simulink model "slturtlesim_control"  (R2021b)
settings: Solver=FixedStepAuto  StartTime=0.0  StopTime=Inf  RelTol=1e-3
undefined symbols (not defined in the file): angular, Call, Function, linear, theta, x, y
libraries: ros2lib x4, simulink x1, mobileRoboticsLib x1
settings Model: Creator=beave  LastModifiedBy=beave
settings OptimizationCC: EnhancedBackFolding=on  PassReuseOutputArgsAs=Individual arguments  ZeroExternalMemoryAtStartup=off  ZeroInternalMemoryAtStartup=off  MaxStackSize=64  OptimizeBlockOrder=speed  DifferentSizesBufferReuse=on  OptimizationCustomize=off  EfficientTunableParamExpr=on
settings DebuggingCC: ParameterTunabilityLossMsg=error
settings SFSimCC: MATLABDynamicMemAlloc=off
settings RTWCC: Description=Embedded Coder  SystemTargetFile=ert.tlc  HardwareBoard=Robot Operating System 2 (ROS 2)  TemplateMakefile=ert_default_tmf  Toolchain=Colcon Tools  TargetLang=C++
settings CodeAppCC: ForceParamTrailComments=on  IgnoreCustomStorageClasses=off  OperatorAnnotations=on  SimulinkDataObjDesc=on  SFDataObjDesc=on  InsertBlockDesc=on
settings ERTTargetCC: CodeInterfacePackaging=C++ class  SupportContinuousTime=on  RootIOFormat=Structure reference

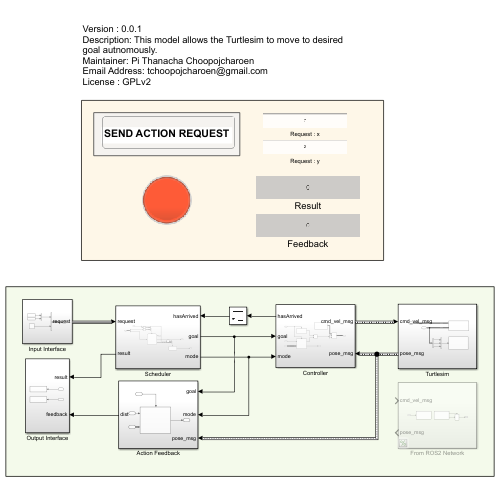
[thumbnail: Simulink's stored preview of the top-level diagram]
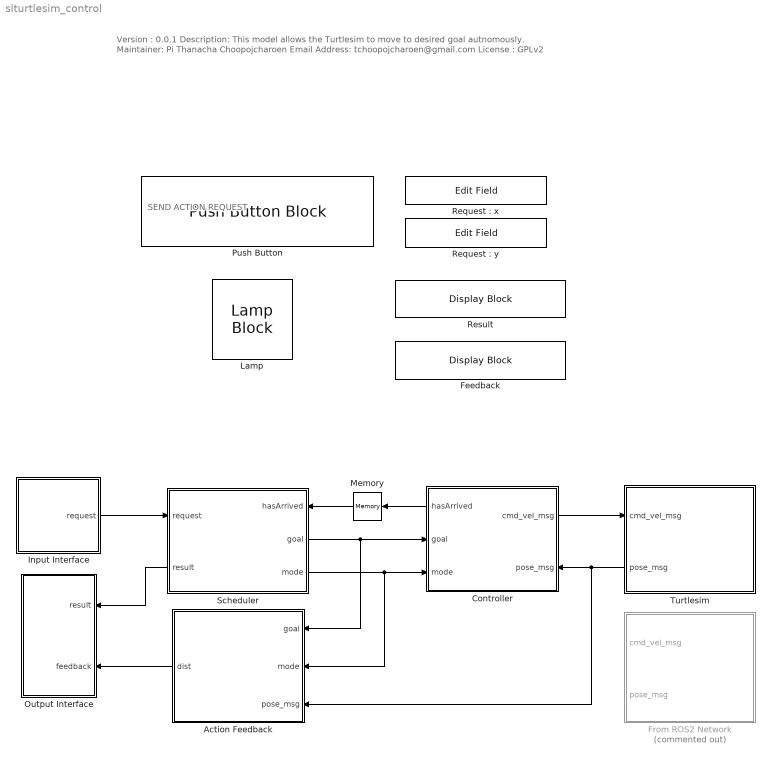
== system slturtlesim_control ==
  note: Version : 0.0.1
      | Description: This model allows the Turtlesim to move to desired goal autnomously.
      | Maintainer: Pi Thanacha Choopojcharoen
      | Email Address: tchoopojcharoen@gmail.com
      | License : GPLv2
  note: SEND ACTION REQUEST
  Action Feedback : Subsystem
      settings: PortSchema="{\"entries\":[{\"content\":{\"sides\":[{\"content\":{\"connectorIds\":[\"Out1\"]},\"type\":\"ConnectorPlacement.EquallySpacedRectSide\",\"uuid\":\"16802256-551c-4223-bfc5-a76a4b41f33f\"},{\"content\":{\"connectorIds\":[\"In1\",\"In2\",\"In3\"],\"side\":\"RIGHT\"},\"type\":\"ConnectorPlacement.EquallySpacedRectSide\",\"uuid\":\"5606428e-27b0-4fd9-928f-2a9a8baead9b\"},{\"content\":{\"connectorIds\":[],\"side\":\"TOP\"},\"type\":\"ConnectorPlacement.EquallySpacedRectSide\",\"uuid\":\"29cf616f-a397-4c6b-9e61-c1bdda273a98\"}]},\"type\":\"ConnectorPlacement.EquallySpacedConnector\",\"uuid\":\"ad2a9b87-c534-416c-adde-7d63bbec43f7\"}],\"packageUris\":[\"http://schema.mathworks.com/mf0/Connector/R2020b\"],\"version\":\"1.0\"}"
  Controller : Subsystem
      settings: PortSchema="{\"entries\":[{\"content\":{\"sides\":[{\"content\":{\"connectorIds\":[\"Out2\",\"In1\",\"In2\"]},\"type\":\"ConnectorPlacement.EquallySpacedRectSide\",\"uuid\":\"038c2229-5bef-4150-bdd4-e0d53c992ca9\"},{\"content\":{\"connectorIds\":[\"Out1\",\"In3\"],\"side\":\"RIGHT\"},\"type\":\"ConnectorPlacement.EquallySpacedRectSide\",\"uuid\":\"f3336771-d94a-4ec8-8106-6e13fcccc0ae\"},{\"content\":{\"connectorIds\":[],\"side\":\"TOP\"},\"type\":\"ConnectorPlacement.EquallySpacedRectSide\",\"uuid\":\"c9d4cbcf-6a2f-41c3-9d97-35a13869506d\"},{\"content\":{\"connectorIds\":[],\"side\":\"BOTTOM\"},\"type\":\"ConnectorPlacement.EquallySpacedRectSide\",\"uuid\":\"fffd547c-1bb9-4cdd-bfe2-128d74787c10\"}]},\"type\":\"ConnectorPlacement.EquallySpacedConnector\",\"uuid\":\"42e11a89-ad8d-483b-9082-68cf3f59b49f\"}],\"packageUris\":[\"http://schema.mathworks.com/mf0/Connector/R2020b\"],\"version\":\"1.0\"}"
  Feedback : DisplayBlock  LabelPosition=Hide  Format=short  Transparency=1
  From ROS2 Network : Subsystem  Commented=on
      settings: PortSchema="{\"entries\":[{\"content\":{\"sides\":[{\"content\":{\"connectorIds\":[\"In1\",\"Out1\"]},\"type\":\"ConnectorPlacement.EquallySpacedRectSide\",\"uuid\":\"f269cb0f-6751-420c-b024-d2e3796ade5b\"},{\"content\":{\"connectorIds\":[],\"side\":\"RIGHT\"},\"type\":\"ConnectorPlacement.EquallySpacedRectSide\",\"uuid\":\"2b43efcf-3102-43c3-9588-0e0fabe7b77d\"},{\"content\":{\"connectorIds\":[],\"side\":\"TOP\"},\"type\":\"ConnectorPlacement.EquallySpacedRectSide\",\"uuid\":\"af694c79-adb9-467b-a06b-a7c95e051029\"}]},\"type\":\"ConnectorPlacement.EquallySpacedConnector\",\"uuid\":\"1952be18-0165-4d1b-9c7c-2327e5c332ed\"}],\"packageUris\":[\"http://schema.mathworks.com/mf0/Connector/R2020b\"],\"version\":\"1.0\"}"
  Input Interface : Subsystem
  Lamp : LampBlock  LabelPosition=Hide
  Memory : Memory  InitialCondition=1
  Output Interface : Subsystem
  Push Button : PushButtonBlock  Opacity=0  IconAlignment=Center  IconColor=On  OffValue=0.000000
  "Request : x" : EditField  LabelPosition=Hide  ShowInitialText=on  Alignment=Center
  "Request : y" : EditField  LabelPosition=Hide  ShowInitialText=on  Alignment=Center
  Result : DisplayBlock  LabelPosition=Hide  Format=short  Transparency=1
  Scheduler : Subsystem
      settings: PortSchema="{\"entries\":[{\"content\":{\"sides\":[{\"content\":{\"connectorIds\":[\"In1\",\"Out3\"]},\"type\":\"ConnectorPlacement.EquallySpacedRectSide\",\"uuid\":\"1630b4b1-4c51-4b39-8ddc-aa89298d57f7\"},{\"content\":{\"connectorIds\":[\"In2\",\"Out1\",\"Out2\"],\"side\":\"RIGHT\"},\"type\":\"ConnectorPlacement.EquallySpacedRectSide\",\"uuid\":\"26eab6e1-3412-432a-b46d-5233f76b34aa\"},{\"content\":{\"connectorIds\":[],\"side\":\"TOP\"},\"type\":\"ConnectorPlacement.EquallySpacedRectSide\",\"uuid\":\"460729cf-3c40-4892-baa8-6e87916f7267\"}]},\"type\":\"ConnectorPlacement.EquallySpacedConnector\",\"uuid\":\"4b48c5f2-6058-4723-aff1-2a33b1e01132\"}],\"packageUris\":[\"http://schema.mathworks.com/mf0/Connector/R2020b\"],\"version\":\"1.0\"}"
  Turtlesim : Subsystem
      settings: PortSchema="{\"entries\":[{\"content\":{\"sides\":[{\"content\":{\"connectorIds\":[\"In1\",\"Out1\"]},\"type\":\"ConnectorPlacement.EquallySpacedRectSide\",\"uuid\":\"f269cb0f-6751-420c-b024-d2e3796ade5b\"},{\"content\":{\"connectorIds\":[],\"side\":\"RIGHT\"},\"type\":\"ConnectorPlacement.EquallySpacedRectSide\",\"uuid\":\"2b43efcf-3102-43c3-9588-0e0fabe7b77d\"},{\"content\":{\"connectorIds\":[],\"side\":\"TOP\"},\"type\":\"ConnectorPlacement.EquallySpacedRectSide\",\"uuid\":\"af694c79-adb9-467b-a06b-a7c95e051029\"}]},\"type\":\"ConnectorPlacement.EquallySpacedConnector\",\"uuid\":\"1952be18-0165-4d1b-9c7c-2327e5c332ed\"}],\"packageUris\":[\"http://schema.mathworks.com/mf0/Connector/R2020b\"],\"version\":\"1.0\"}"
  wires:
  Controller/2(hasArrived) -> Memory/1
  Scheduler/1(goal) -> Action Feedback/1(goal), Controller/1(goal)
  Scheduler/2(mode) -> Action Feedback/2(mode), Controller/2(mode)
  Memory/1 -> Scheduler/2(hasArrived)
  Turtlesim/1(pose_msg) -> Action Feedback/3(pose_msg), Controller/3(pose_msg)
  Controller/1(cmd_vel_msg) -> Turtlesim/1(cmd_vel_msg)
  Scheduler/3(result) -> Output Interface/1(result)
  Action Feedback/1(dist) -> Output Interface/2(feedback)
  Input Interface/1(request) -> Scheduler/1(request)

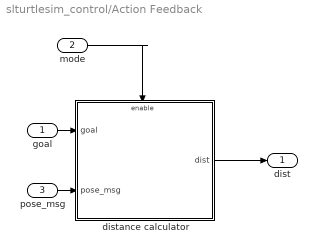
== system slturtlesim_control/Action Feedback ==
  goal : Inport
  mode : Inport  Port=2
  pose_msg : Inport  Port=3
  distance calculator : Subsystem
  dist : Outport
  wires:
  distance calculator/1(dist) -> dist/1
  pose_msg/1 -> distance calculator/2(pose_msg)
  goal/1 -> distance calculator/1(goal)
  mode/1 -> distance calculator/Enable

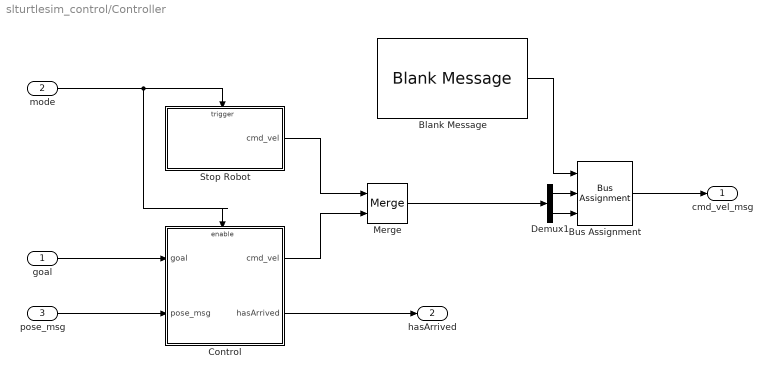
== system slturtlesim_control/Controller ==
  goal : Inport
  mode : Inport  Port=2
  pose_msg : Inport  Port=3
  Blank Message : ros2lib/Blank Message  messageClass=Message  entityType=geometry_msgs/Twist  messageType=geometry_msgs/Twist  SampleTime=inf
      settings: SourceProductBaseCode=RR
  Bus Assignment : BusAssignment  AssignedSignals=linear.x,angular.z
  Control : Subsystem
  Demux1 : Demux  Outputs=2
  Merge : Merge  InitialOutput=[0;0]
  Stop Robot : Subsystem
  cmd_vel_msg : Outport
  hasArrived : Outport  Port=2
  wires:
  pose_msg/1 -> Control/2(pose_msg)
  Control/2(hasArrived) -> hasArrived/1
  goal/1 -> Control/1(goal)
  mode/1 -> Control/Enable, Stop Robot/Trigger
  Control/1(cmd_vel) -> Merge/2
  Stop Robot/1(cmd_vel) -> Merge/1
  Blank Message/1 -> Bus Assignment/1
  Demux1/1 -> Bus Assignment/2
  Demux1/2 -> Bus Assignment/3
  Merge/1 -> Demux1/1
  Bus Assignment/1 -> cmd_vel_msg/1

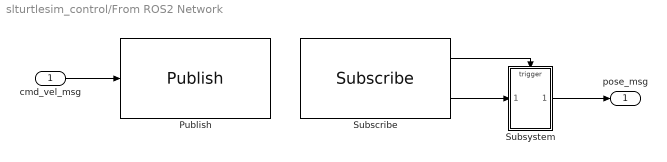
== system slturtlesim_control/From ROS2 Network ==
  cmd_vel_msg : Inport
  Publish : ros2lib/Publish  topicSource=Specify your own  topic=/turtle1/cmd_vel  messageType=geometry_msgs/Twist  QOSHistory=Keep last  QOSDepth=1  QOSReliability=Reliable  QOSDurability=Volatile
      settings: SourceProductBaseCode=RR
  Subscribe : ros2lib/Subscribe  topicSource=Select from ROS network  topic=/turtle1/pose  messageType=geometry_msgs/Point  sampleTime=-1  QOSHistory=Keep last  QOSDepth=1  QOSReliability=Reliable  QOSDurability=Volatile
      settings: SourceProductBaseCode=RR
  Subsystem : Subsystem
  pose_msg : Outport
  wires:
  cmd_vel_msg/1 -> Publish/1
  Subsystem/1(Out1) -> pose_msg/1
  Subscribe/1 -> Subsystem/Trigger
  Subscribe/2 -> Subsystem/1(In1)

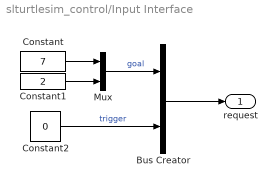
== system slturtlesim_control/Input Interface ==
  Bus Creator : BusCreator  Inputs=2
  Constant : Constant  Value=7
  Constant1 : Constant  Value=2
  Constant2 : Constant  Value=0
  Mux : Mux  Inputs=2
  request : Outport
  wires:
  Mux/1 -> Bus Creator/1  "goal"
  Constant1/1 -> Mux/2
  Constant/1 -> Mux/1
  Constant2/1 -> Bus Creator/2  "trigger"
  Bus Creator/1 -> request/1

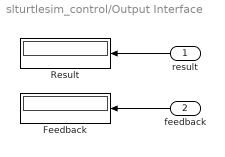
== system slturtlesim_control/Output Interface ==
  result : Inport
  feedback : Inport  Port=2
  Feedback : Display
  Result : Display
  wires:
  result/1 -> Result/1
  feedback/1 -> Feedback/1

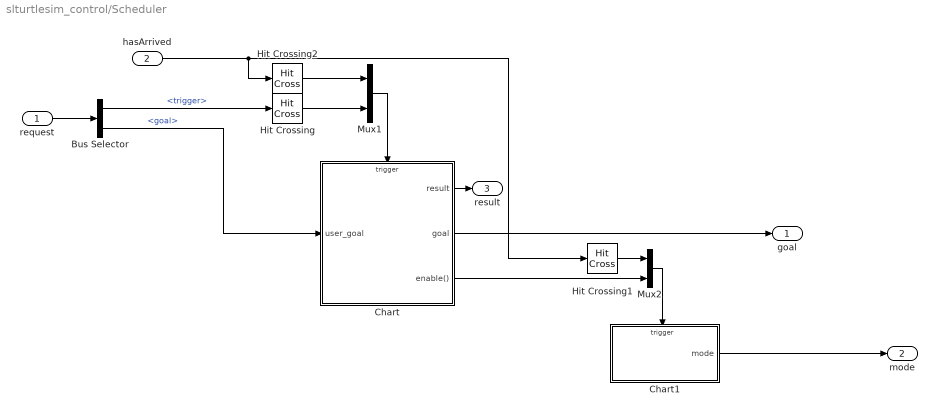
== system slturtlesim_control/Scheduler ==
  request : Inport
  hasArrived : Inport  Port=2
  Bus Selector : BusSelector  OutputSignals=trigger,goal
  Chart : Stateflow chart  TreatAsAtomicUnit=on
  Chart1 : Stateflow chart  TreatAsAtomicUnit=on
  Hit Crossing : HitCross  HitCrossingDirection=rising  HitCrossingOutputType=Function-Call
  Hit Crossing1 : HitCross  HitCrossingDirection=rising  HitCrossingOutputType=Function-Call
  Hit Crossing2 : HitCross  HitCrossingDirection=rising  HitCrossingOutputType=Function-Call
  Mux1 : Mux  Inputs=2
  Mux2 : Mux  Inputs=2
  goal : Outport
  mode : Outport  Port=2
  result : Outport  Port=3
  wires:
  Chart/2(goal) -> goal/1
  Mux1/1 -> Chart/Trigger
  hasArrived/1 -> Hit Crossing1/1, Hit Crossing2/1
  Chart/3(enable()) -> Mux2/2
  Hit Crossing/1 -> Mux1/2
  Bus Selector/2 -> Chart/1(user_goal)  "<goal>"
  Hit Crossing1/1 -> Mux2/1
  Mux2/1 -> Chart1/Trigger
  Hit Crossing2/1 -> Mux1/1
  Bus Selector/1 -> Hit Crossing/1  "<trigger>"
  Chart/1(result) -> result/1
  Chart1/1(mode) -> mode/1
  request/1 -> Bus Selector/1

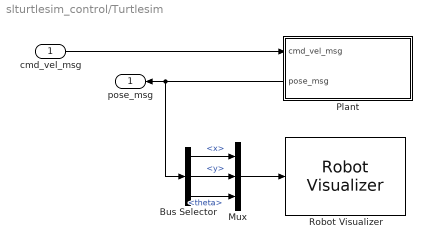
== system slturtlesim_control/Turtlesim ==
  cmd_vel_msg : Inport
  Bus Selector : BusSelector  OutputSignals=x,y,theta
  Mux : Mux  Inputs=3
  Plant : Subsystem
      settings: PortSchema="{\"entries\":[{\"content\":{\"sides\":[{\"content\":{\"connectorIds\":[\"In1\",\"Out1\"]},\"type\":\"ConnectorPlacement.EquallySpacedRectSide\",\"uuid\":\"6cc3d191-8b41-43a3-8d7e-fbb38f5f3909\"},{\"content\":{\"connectorIds\":[],\"side\":\"RIGHT\"},\"type\":\"ConnectorPlacement.EquallySpacedRectSide\",\"uuid\":\"02a725d1-914e-48c3-8213-963338e78503\"},{\"content\":{\"connectorIds\":[],\"side\":\"TOP\"},\"type\":\"ConnectorPlacement.EquallySpacedRectSide\",\"uuid\":\"a9769afc-f0de-40ec-971f-b36fa9ae13e3\"}]},\"type\":\"ConnectorPlacement.EquallySpacedConnector\",\"uuid\":\"c85e1385-84c4-4576-8165-8301e6039802\"}],\"packageUris\":[\"http://schema.mathworks.com/mf0/Connector/R2020b\"],\"version\":\"1.0\"}"
  Robot Visualizer : mobileRoboticsLib/Environments/Robot Visualizer  Priority=99  robotRadius=0  showTrajectory=on  hasWaypoints=off  hasLidar=off  sensorOffset=[ 0 0 ]  scanAngles=0  hasObjDetector=off  objDetectorOffset=[ 0, 0 ]  objDetectorAngle=0  objDetectorFOV=0  objDetectorMaxRange=0  objectColors=0  objectMarkers=s
      settings: SourceProductName=Ground Vehicles Library
  pose_msg : Outport
  wires:
  Bus Selector/2 -> Mux/2  "<y>"
  Bus Selector/3 -> Mux/3  "<theta>"
  Mux/1 -> Robot Visualizer/1
  cmd_vel_msg/1 -> Plant/1(cmd_vel_msg)
  Bus Selector/1 -> Mux/1  "<x>"
  Plant/1(pose_msg) -> Bus Selector/1, pose_msg/1

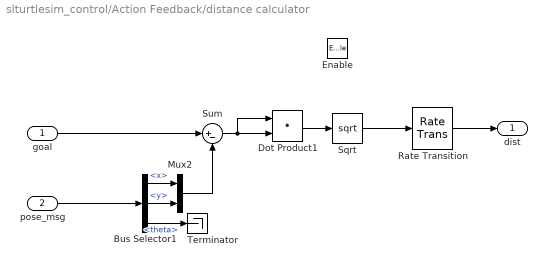
== system slturtlesim_control/Action Feedback/distance calculator ==
  goal : Inport
  pose_msg : Inport  Port=2
  Enable : EnablePort
  Bus Selector1 : BusSelector  OutputSignals=x,y,theta
  Dot Product1 : DotProduct  InputSameDT=on  OutDataTypeStr=Inherit: Inherit via internal rule
  Mux2 : Mux  Inputs=2
  Rate Transition : RateTransition  OutPortSampleTime=0.1
  Sqrt : Sqrt  SaturateOnIntegerOverflow=on
  Sum : Sum  Inputs=|+-
  Terminator : Terminator
  dist : Outport
  wires:
  pose_msg/1 -> Bus Selector1/1
  Bus Selector1/1 -> Mux2/1  "<x>"
  Mux2/1 -> Sum/2
  goal/1 -> Sum/1
  Sum/1 -> Dot Product1/2, Dot Product1/1
  Dot Product1/1 -> Sqrt/1
  Bus Selector1/3 -> Terminator/1  "<theta>"
  Bus Selector1/2 -> Mux2/2  "<y>"
  Sqrt/1 -> Rate Transition/1
  Rate Transition/1 -> dist/1

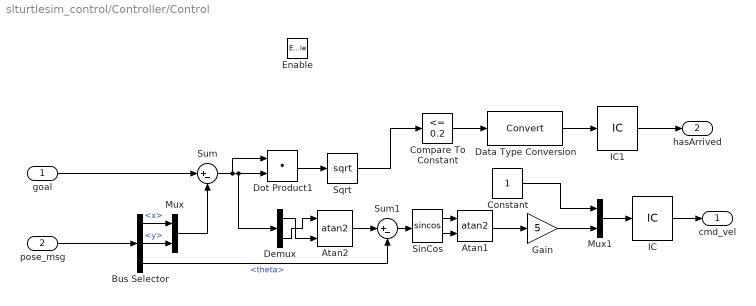
== system slturtlesim_control/Controller/Control ==
  goal : Inport
  pose_msg : Inport  Port=2
  Enable : EnablePort
  Atan1 : Trigonometry  Operator=atan2
  Atan2 : Trigonometry  Operator=atan2
  Bus Selector : BusSelector  OutputSignals=x,y,theta
  Compare To Constant : simulink/Logic and Bit Operations/Compare To Constant  relop=<=  const=0.2  OutDataTypeStr=boolean
  Constant : Constant
  Data Type Conversion : DataTypeConversion
  Demux : Demux  Outputs=2
  Dot Product1 : DotProduct  InputSameDT=on  OutDataTypeStr=Inherit: Inherit via internal rule
  Gain : Gain  Gain=5
  IC : InitialCondition  Value=[0;0]
  IC1 : InitialCondition
  Mux : Mux  Inputs=2
  Mux1 : Mux  Inputs=2
  SinCos : Trigonometry  Operator=sincos
  Sqrt : Sqrt  SaturateOnIntegerOverflow=on
  Sum : Sum  Inputs=|+-
  Sum1 : Sum  Inputs=|+-
  cmd_vel : Outport
  hasArrived : Outport  Port=2
  wires:
  Constant/1 -> Mux1/1
  Demux/1 -> Atan2/2
  SinCos/1 -> Atan1/1
  Gain/1 -> Mux1/2
  Bus Selector/2 -> Mux/2  "<y>"
  Demux/2 -> Atan2/1
  Atan1/1 -> Gain/1
  Bus Selector/1 -> Mux/1  "<x>"
  Atan2/1 -> Sum1/1
  Bus Selector/3 -> Sum1/2  "<theta>"
  Sum/1 -> Dot Product1/2, Demux/1, Dot Product1/1
  SinCos/2 -> Atan1/2
  Sum1/1 -> SinCos/1
  Mux/1 -> Sum/2
  pose_msg/1 -> Bus Selector/1
  goal/1 -> Sum/1
  Mux1/1 -> IC/1
  IC/1 -> cmd_vel/1
  Sqrt/1 -> Compare To Constant/1
  Compare To Constant/1 -> Data Type Conversion/1
  Dot Product1/1 -> Sqrt/1
  IC1/1 -> hasArrived/1
  Data Type Conversion/1 -> IC1/1

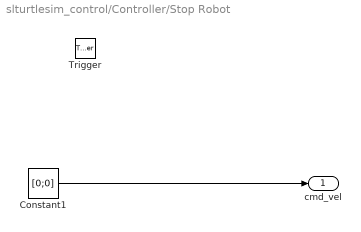
== system slturtlesim_control/Controller/Stop Robot ==
  Trigger : TriggerPort  TriggerType=falling  VariantControl=(inherit)  PortDimensions=1
  Constant1 : Constant  Value=[0;0]
  cmd_vel : Outport
  wires:
  Constant1/1 -> cmd_vel/1

== system slturtlesim_control/From ROS2 Network/Subsystem ==
  In1 : Inport
  Trigger : TriggerPort  VariantControl=(inherit)  PortDimensions=1
  Out1 : Outport
  wires:
  In1/1 -> Out1/1

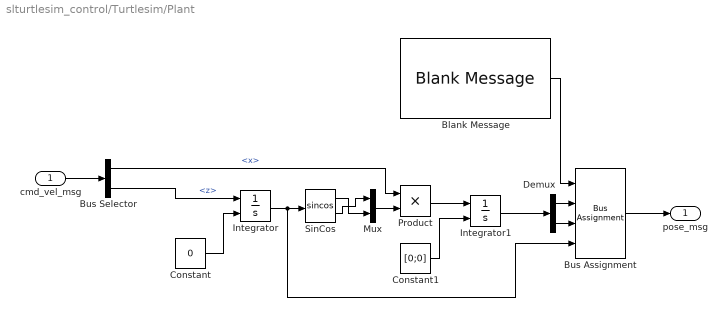
== system slturtlesim_control/Turtlesim/Plant ==
  cmd_vel_msg : Inport
  Blank Message : ros2lib/Blank Message  messageClass=Message  entityType=geometry_msgs/Pose2D  messageType=geometry_msgs/Pose2D  SampleTime=inf
      settings: SourceProductBaseCode=RR
  Bus Assignment : BusAssignment  AssignedSignals=x,y,theta
  Bus Selector : BusSelector  OutputSignals=linear.x,angular.z
  Constant : Constant  Value=0
  Constant1 : Constant  Value=[0;0]
  Demux : Demux  Outputs=2
  Integrator : Integrator  InitialConditionSource=external
  Integrator1 : Integrator  InitialConditionSource=external
  Mux : Mux  Inputs=2
  Product : Product
  SinCos : Trigonometry  Operator=sincos
  pose_msg : Outport
  wires:
  Bus Assignment/1 -> pose_msg/1
  Integrator/1 -> Bus Assignment/4, SinCos/1
  Product/1 -> Integrator1/1
  SinCos/2 -> Mux/1
  cmd_vel_msg/1 -> Bus Selector/1
  Demux/1 -> Bus Assignment/2
  Mux/1 -> Product/2
  Blank Message/1 -> Bus Assignment/1
  Integrator1/1 -> Demux/1
  Constant1/1 -> Integrator1/2
  SinCos/1 -> Mux/2
  Demux/2 -> Bus Assignment/3
  Bus Selector/1 -> Product/1  "<x>"
  Bus Selector/2 -> Integrator/1  "<z>"
  Constant/1 -> Integrator/2

== stateflow chart slturtlesim_control/Scheduler/Chart1 ==
  settings: executeAtInitialization=1
  state IDLE
  state RUN
  (default) -> IDLE : {mode = 0}
  IDLE -> RUN : enable{mode = 1;}
  RUN -> IDLE : hasArrived{mode = 0;}
  data: mode output
  events: hasArrived input FUNCTION_CALL_EVENT; enable input FUNCTION_CALL_EVENT

== stateflow chart slturtlesim_control/Scheduler/Chart ==
  settings: executeAtInitialization=1
  state IDLE
  state WAIT
  (default) -> IDLE : {goal = [0;0];}
  IDLE -> WAIT : execute/{t_0 = t;goal = user_goal;send(enable);disp('enable!!')}
  WAIT -> IDLE : hasReached{result = t-t_0}
  data: t_0 local; result output; goal output; user_goal input
  events: hasReached input FUNCTION_CALL_EVENT; execute input FUNCTION_CALL_EVENT; enable output FUNCTION_CALL_EVENT
